simulink model "PlantFunc"  (R2020a)
settings: Solver=VariableStepAuto  StartTime=0.0  StopTime=10.0  RelTol=1e-3
libraries: simulink x1
settings Model: Creator=ivanholodilin  LastModifiedBy=ivanholodilin

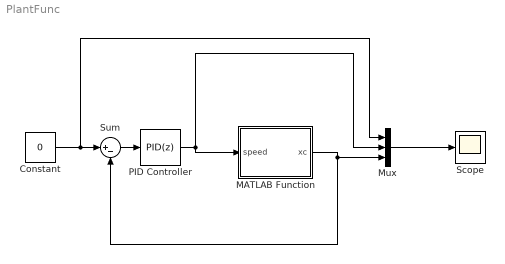
== system PlantFunc ==
  Constant : Constant  Value=0
  MATLAB Function : MATLAB Function  TreatAsAtomicUnit=on
  Mux : Mux  Inputs=3
  PID Controller : simulink/Continuous/PID Controller  Controller=PID  Form=Parallel  TimeDomain=Discrete-time  UseExternalTs=off  SampleTime=-1  IntegratorMethod=Forward Euler  FilterMethod=Forward Euler  ControllerParametersSource=internal  P=24  I=1  D=8  UseFilter=on  N=100  TunerSelectOption=Transfer Function Based (PID Tuner App)  InitialConditionSource=internal  InitialConditionForIntegrator=0  InitialConditionForFilter=0  DifferentiatorICPrevScaledInput=0  ExternalReset=none  TrackingMode=off  Kt=1  LimitOutput=on  UpperSaturationLimit=10  LowerSaturationLimit=-10  LinearizeAsGain=on  AntiWindupMode=back-calculation  Kb=1  POutMin=[]  POutMax=[]  IOutMin=[]  IOutMax=[]  DOutMin=[]  DOutMax=[]  NOutMin=[]  NOutMax=[]  SumOutMin=[]  SumOutMax=[]  SaturationOutMin=[]  SaturationOutMax=[]  PParamMin=[]  PParamMax=[]  IParamMin=[]  IParamMax=[]  DParamMin=[]  DParamMax=[]  NParamMin=[]  NParamMax=[]  KbParamMin=[]  KbParamMax=[]  KtParamMin=[]  KtParamMax=[]  KbOutMin=[]  KbOutMax=[]  KtOutMin=[]  KtOutMax=[]  IntegratorOutMin=[]  IntegratorOutMax=[]  FilterOutMin=[]  FilterOutMax=[]  SumI1OutMin=[]  SumI1OutMax=[]  SumI2OutMin=[]  SumI2OutMax=[]  SumI3OutMin=[]  SumI3OutMax=[]  SumI4OutMin=[]  SumI4OutMax=[]  SumDOutMin=[]  SumDOutMax=[]  DifferentiatorOutMin=[]  DifferentiatorOutMax=[]  FilterDiffOutCoefMin=[]  FilterDiffOutCoefMax=[]  ReciprocalOutMin=[]  ReciprocalOutMax=[]  SumDenOutMin=[]  SumDenOutMax=[]  SumNumOutMin=[]  SumNumOutMax=[]  DivideOutMin=[]  DivideOutMax=[]  UdiffTsProdOutMin=[]  UdiffTsProdOutMax=[]  NTsProdOutMin=[]  NTsProdOutMax=[]  UintegralTsProdOutMin=[]  UintegralTsProdOutMax=[]  UngainTsProdOutMin=[]  UngainTsProdOutMax=[]  IntegratorContinuousStateAttributes=''  IntegratorStateMustResolveToSignalObject=off  IntegratorRTWStateStorageClass=Auto  FilterContinuousStateAttributes=''  FilterStateMustResolveToSignalObject=off  FilterRTWStateStorageClass=Auto  ParallelPVariant=InternalParameters  IdealPVariant=Disabled  IVariant=InternalParameters  DVariant=InternalParameters  IntegratorVariant=Discrete  SatVariant=Enabled  AWVariant=BackCalculation  PCopyVariant=Disabled  TRVariant=Disabled  FdbkBlocksVariant=Forward  IdealPFdbkVariant=Disabled  SatFdbkVariant=Disabled  DerivativeFilterVariant=ForwardEulerFilter  NVariant=InternalParameters  NCopyVariant=Disabled  FilterICVariant=InternalICsFilter  IntegratorICVariant=InternalICs  ExternalResetVariant=Disabled  TRSumVariant=Passthrough  SumFdbkVariant=Disabled  SumVariant=Sum_PID  TsampFilterVariant=InternalTs  TsampNgainVariant=Passthrough  TsampIntegralVariant=Passthrough
  Scope : Scope
  Sum : Sum  Inputs=|+-
  wires:
  Constant/1 -> Mux/1, Sum/1
  Sum/1 -> PID Controller/1
  PID Controller/1 -> MATLAB Function/1(speed), Mux/2
  MATLAB Function/1(xc) -> Sum/2, Mux/3
  Mux/1 -> Scope/1

== matlab function PlantFunc/MATLAB Function ==
  data: speed input; xc output
function xc = fcn(speed)
 
% Initialization Parameters
server_ip = '127.0.0.1';     % IP address of the Unity Server
server_port = 55001;         % Server Port of the Unity Sever
% The Client obj that is created is the connection to the server
% TCPInit func;

TCP_Handle = tcpclient(server_ip,server_port);
fprintf(1,"Connected to server\n");
 
% MotionVer func
int = 7; % 0-img, 1-transform, 2-get position, 3-mode, 4-laser, 5-set position,
% 6 - motion vertical, 7 - motion horizontal
write(TCP_Handle,single([int,speed]));
 
ocam_model = 1;
 
% mapping configuration
camX = 0; % Camera parameters
camY = 0; % Camera parameters
camZ = 0; % Camera parameters
lasX = 0; % Laser Plane parameters
lasY = 0; % Laser Plane parameters
las_dist = 666; % Laser Plane parameters
 
% Initialization Parameters
height = 1920; % image size
width = 1920; % image size
 
 
 
figure;
% GetImage func
write(TCP_Handle,single([0,height,width])); % 0-img, 1-transform, 2-both img&transform
%Get image data
data = read(TCP_Handle,height*width*3);
%Organizing image data
imagetmp = uint8(zeros(width,height,3));
image = uint8(zeros(height,width,3));
r = uint8(zeros(height,width));
g = uint8(zeros(height,width));
b = uint8(zeros(height,width));
r = data(1:3:width*height*3);
g = data(2:3:width*height*3);
b = data(3:3:width*height*3);
for y = 1:height
    for x = 1:width
        imagetmp(x,y,1) = r((y-1)*width+x);
        imagetmp(x,y,2) = g((y-1)*width+x);
        imagetmp(x,y,3) = b((y-1)*width+x);
    end
end
image = uint8(imrotate(imagetmp,90));
pause(0.15);
imshow(image);
 
 
 
% Mapping
% las_segm_red func
[height, width, planes] = size(image);
rgb = reshape(image, height, width * planes);
imagesc(rgb);  
% visualize RGB planes 
r = image(:, :, 1);             % red channel
g = image(:, :, 2);             % green channel
b = image(:, :, 3);             % blue channel
threshold = 100;                % threshold value
imagesc(r < threshold);         % display the binarized image
blueness = double(r) - max(double(g), double(b));
imagesc(blueness);              % visualize RGB planes
 mask = blueness < val;
imagesc(mask);
labels = bwlabel(mask);
id = labels(200, 200);
las = (labels == id);
imagesc(las); 
J = imcomplement(las);
BW = im2bw(J,0.4);
 
 
 
% mapping func
[height,width] = size(BW);
Z=las_dist;
a = 1;
% x1=[];
% y1=[];
x1 = zeros(1,height);
y1 = zeros(1,height);
t = [0;0;Z];
% compose_rotation func
X = eye(3,3);
Y = eye(3,3);
Z = eye(3,3);
X(2,2) = cosd(lasX);
X(2,3) = -sind(lasX);
X(3,2) = sind(lasX);
X(3,3) = cosd(lasX);
Y(1,1) = cosd(lasY);
Y(1,3) = sind(lasY);
Y(3,1) = -sind(lasY);
Y(3,3) = cosd(lasY);
Z(1,1) = cosd(0);
Z(1,2) = -sind(0);
Z(2,1) = sind(0);
Z(2,2) = cosd(0);
r = Z*Y*X;
 
% compose_rotation func
X = eye(3,3);
Y = eye(3,3);
Z = eye(3,3);
X(2,2) = cosd(-camX);
X(2,3) = -sind(-camX);
X(3,2) = sind(-camX);
X(3,3) = cosd(-camX);
Y(1,1) = cosd(-camY);
Y(1,3) = sind(-camY);
Y(3,1) = -sind(-camY);
Y(3,3) = cosd(-camY);
Z(1,1) = cosd(camZ);
Z(1,2) = -sind(camZ);
Z(2,1) = sind(camZ);
Z(2,2) = cosd(camZ);
r_ = Z*Y*X;
 
r = r_*[r(:,1),r(:,2),t];

ss = [-6.135313575065034e+02;0;6.074792332342159e-04;-1.755490735537311e-07;2.449842232995912e-10];
x_c = 9.605462213569594e+02;
y_c = 9.606391421585625e+02;
width = 1920;
height = 1920;
c = 0.999956539600431;
d = 2.132336434678594e-06;
e = -8.627881999764250e-06;
A = [c,d;
     e,1];
for i=1:height      % working image region
    for j=1:width
        if BW(i,j)>0
            m=[i;j];       % image pixels
            % cam2world func
            n_points = size(m,2);
            T = [x_c;y_c]*ones(1,n_points);
            m = A^-1*(m-T);
            % getpoint func;
            M = [m(1,:) ; m(2,:) ; polyval(ss(end:-1:1),sqrt(m(1,:).^2+m(2,:).^2)) ];      
            
            a1 = M(1)*r(2,1)-M(2)*r(1,1);
            b1 = M(1)*r(2,2)-M(2)*r(1,2);
            c1 = M(1)*r(2,3)-M(2)*r(1,3);
            a2 = M(3)*r(1,1)-M(1)*r(3,1);
            b2 = M(3)*r(1,2)-M(1)*r(3,2);
            c2 = M(3)*r(1,3)-M(1)*r(3,3);
 
            Y = (a2*c1-a1*c2)/(a1*b2-a2*b1);
            X = (-c1-b1*Y)/a1;               
        
            y1(a)=X;
            x1(a)=-Y; 
            a=a+1;
        end
    end
end
 
 
% Finally figure:
figure;
scatter(x1,y1,5,'filled'); % Laser intersections, first image
hold on;
% Reference circle
% circfit func;  
x1=x1(:); y1=y1(:);
a=[x1 y1 ones(size(x1))]\[-(x1.^2+y1.^2)];
xc = -.5*a(1);
yc = -.5*a(2);
R  =  sqrt((a(1)^2+a(2)^2)/4-a(3));

th = 0:pi/50:2*pi;
xunit = R * cos(th) + xc;
yunit = R * sin(th) + yc;
plot(xunit, yunit);
plot(xc, yc, 'o');
grid on;
axis equal
 
%Close Gracefully
fprintf(1,"Disconnected from server\n");
R
end
